simulink model "untitled"  (R2018a)
settings: Solver=VariableStepAuto  StartTime=0.0  StopTime=10.0  RelTol=1e-3
libraries: cstblocks x1, mpclib x1
settings Model: Creator=ja  LastModifiedBy=ja

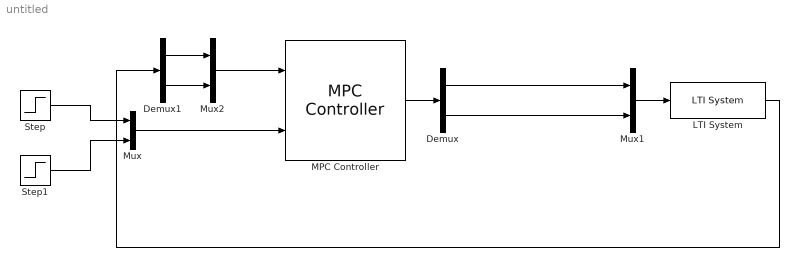
== system untitled ==
  Demux : Demux  Outputs=2
  Demux1 : Demux  Outputs=2
  LTI System : cstblocks/LTI System  sys=Plant  IC=[]
  MPC Controller : mpclib/MPC Controller  SCDEnableBlockLinearizationSpecification=on  is_multiple=0  enable_value=0  return_u0=off  updateMPCinCallerWorkspace=on  ref_from_ws=off  ref_signal_name=[]  ref_preview=off  md_from_ws=off  md_signal_name=[]  md_preview=off  from_project=off  project_file=MPCtask.mat  md_inport=off  mv_inport=off  cost_outport=off  return_sequence=off  return_qpstatus=off  return_state=off  state_inport=off  lims_inport=off  cc_inport=off  ywt_inport=off  is_designfromscratch=0  uwt_inport=off  duwt_inport=off  rhoeps_inport=off  uref_inport=off  n_ts=1  n_p=10  n_mv=2  n_md=1  n_ud=0  n_mo=2  n_uo=0  BlockDataType=double  SampleTimeInherited=off  switch_inport=off
  Mux : Mux  Inputs=2
  Mux1 : Mux  Inputs=2
  Mux2 : Mux  Inputs=2
  Step : Step  After=10  SampleTime=0
  Step1 : Step  Time=10  SampleTime=0
  wires:
  Mux/1 -> MPC Controller/2
  Step1/1 -> Mux/2
  Step/1 -> Mux/1
  MPC Controller/1 -> Demux/1
  Mux1/1 -> LTI System/1
  Demux/2 -> Mux1/2
  Demux/1 -> Mux1/1
  Mux2/1 -> MPC Controller/1
  Demux1/1 -> Mux2/1
  Demux1/2 -> Mux2/2
  LTI System/1 -> Demux1/1
